simulink model "ukol_9_integr_model"  (R2017a)
settings: Solver=VariableStepAuto  StartTime=0.0  StopTime=30  MaxStep=1e-3  RelTol=1e-3
values from neighbouring files (symbols this model uses):
  A = [0 1; -1.44 -0.36]    [ukol_5_script.m]
  B = [0; 1]    [ukol_5_script.m]
  C_1 = [7.2 0]    [ukol_5_script.m]
  D = [0; 0]    [ukol_5_script.m]    (also in ukol_8_script.m = 0; ukol_9_script.m)
  k1_2 = 3.765    [ukol_5_script.m]
  k2_2 = 2.363    [ukol_5_script.m]
  kI = 0.523    [ukol_5_script.m]
  L = [0.505555; 0.173555]    [ukol_8_script.m]
settings Model: Creator=tomas  LastModifiedBy=tomas

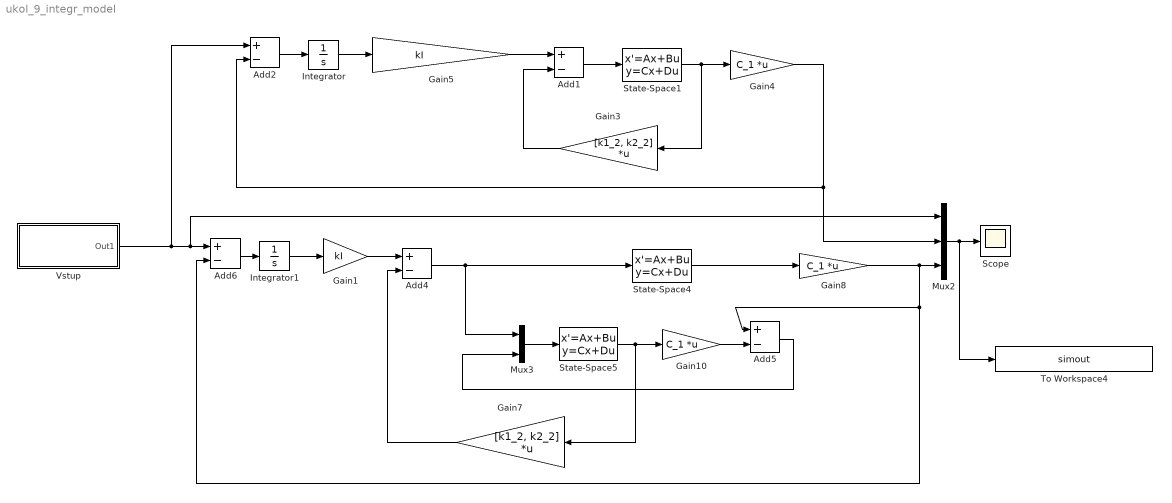
== system ukol_9_integr_model ==
  Add{1..2,4..6} (5 alike) : Sum  Inputs=+-
  Gain1 : Gain  Gain=kI
  Gain10 : Gain  Gain=C_1  Multiplication=Matrix(K*u)
  Gain3 : Gain  Gain=[k1_2, k2_2]  Multiplication=Matrix(K*u)
  Gain4 : Gain  Gain=C_1  Multiplication=Matrix(K*u)
  Gain5 : Gain  Gain=kI
  Gain7 : Gain  Gain=[k1_2, k2_2]  Multiplication=Matrix(K*u)
  Gain8 : Gain  Gain=C_1  Multiplication=Matrix(K*u)
  Integrator : Integrator
  Integrator1 : Integrator
  Mux2 : Mux  Inputs=3
  Mux3 : Mux  Inputs=2
  Scope : Scope
  State-Space1 : StateSpace  A=A  B=B  C=[1 0; 0 1]  D=D  X0=0
  State-Space4 : StateSpace  A=A  B=B  C=[1 0; 0 1]  D=D  X0=0
  State-Space5 : StateSpace  A=A  B=[B L]  C=[1 0; 0 1]  D=[0 0; 0 0]  X0=[0.3;-0.2]
  To Workspace4 : ToWorkspace  VariableName=simout  SaveFormat=Timeseries  SampleTime=-1
  "Vstup " : Subsystem
  wires:
  Add5/1 -> Mux3/2
  Mux2/1 -> To Workspace4/1, Scope/1
  State-Space4/1 -> Gain8/1
  Gain8/1 -> Add6/2, Add5/1, Mux2/3
  Mux3/1 -> State-Space5/1
  State-Space5/1 -> Gain10/1, Gain7/1
  Add4/1 -> State-Space4/1, Mux3/1
  Gain10/1 -> Add5/2
  "Vstup "/1(Out1) -> Add2/1, Add6/1, Mux2/1
  Gain7/1 -> Add4/2
  Add1/1 -> State-Space1/1
  Gain5/1 -> Add1/1
  Add2/1 -> Integrator/1
  Integrator/1 -> Gain5/1
  Gain4/1 -> Mux2/2, Add2/2
  State-Space1/1 -> Gain3/1, Gain4/1
  Gain3/1 -> Add1/2
  Gain1/1 -> Add4/1
  Integrator1/1 -> Gain1/1
  Add6/1 -> Integrator1/1

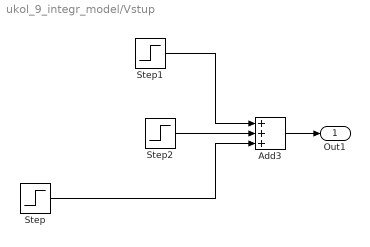
== system ukol_9_integr_model/Vstup  ==
  Add3 : Sum  Inputs=+++
  Step : Step  SampleTime=0
  Step1 : Step  Time=10  After=-4  SampleTime=0
  Step2 : Step  Time=20  After=8  SampleTime=0
  Out1 : Outport
  wires:
  Step2/1 -> Add3/2
  Step/1 -> Add3/3
  Step1/1 -> Add3/1
  Add3/1 -> Out1/1
